simulink model "moore_mp3"  (R2024a)
settings: Solver=FixedStepDiscrete  StartTime=0.0  StopTime=inf  RelTol=1e-3  EnableMultiTasking=on
settings Model: Creator=nunkesser  LastModifiedBy=nunkesser
settings SolverCC: AlgebraicLoopSolver=TrustRegion
settings DataIOCC: LimitDataPoints=on  SaveFormat=Array  ReturnWorkspaceOutputs=off
settings OptimizationCC: LifeSpan=inf
settings DebuggingCC: SolverPrmCheckMsg=warning  UnconnectedInputMsg=warning  UnconnectedOutputMsg=warning  UnconnectedLineMsg=warning  SFUnexpectedBacktrackingDiag=warning  SFNoUnconditionalDefaultTransitionDiag=warning  SFExecutionAtInitializationDiag=none  ArithmeticOperatorsInVariantConditions=warning
settings HardwareCC: ProdBitPerPointer=32  ProdBitPerSizeT=32  ProdBitPerPtrDiffT=32  ProdLargestAtomicFloat=None  ProdIntDivRoundTo=Undefined  ProdEndianess=Unspecified  ProdWordSize=32  ProdHWDeviceType=32-bit Generic
settings ModelReferenceCC: PropagateSignalLabelsOutOfModel=off
settings SFSimCC: SimUseLocalCustomCode=off  CustomCodeUndefinedFunction=UseInterfaceOnly
settings RTWCC: RTWUseLocalCustomCode=off  GPUComputeCapability=3.5
settings CodeAppCC: StateflowObjectComments=on
settings GRTTargetCC: TargetLangStandard=C89/C90 (ANSI)
settings ConfigComp: CovMetricSettings=dw  CovSaveCumulativeToWorkspaceVar=on  CovSaveSingleToWorkspaceVar=on  CovExternalEMLEnable=off  CovSFcnEnable=off

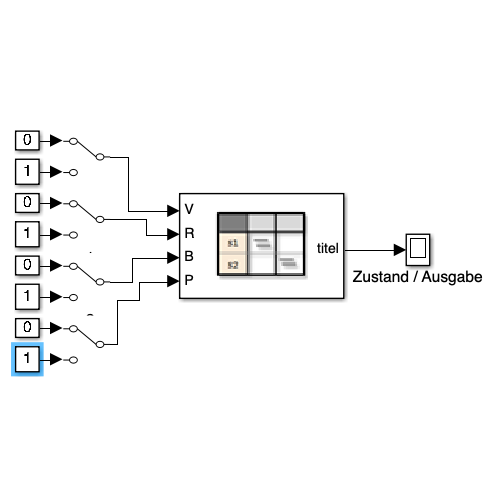
[thumbnail: Simulink's stored preview of the top-level diagram]
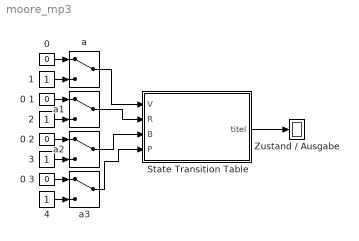
== system moore_mp3 ==
  0 {,1..3} (4 alike) : Constant  Value=0  OutDataTypeStr=boolean
  {1..4} (4 alike) : Constant  OutDataTypeStr=boolean
  State Transition Table : State Transition Table  TreatAsAtomicUnit=on
  Zustand / Ausgabe : Display
  a{,1..3} (4 alike) : ManualSwitch
  wires:
  1/1 -> a/2
  "0 "/1 -> a/1
  a/1 -> State Transition Table/1(V)
  2/1 -> a1/2
  0 1/1 -> a1/1
  a1/1 -> State Transition Table/2(R)
  3/1 -> a2/2
  0 2/1 -> a2/1
  a2/1 -> State Transition Table/3(B)
  4/1 -> a3/2
  0 3/1 -> a3/1
  a3/1 -> State Transition Table/4(P)
  State Transition Table/1(titel) -> Zustand / Ausgabe/1

== stateflow chart moore_mp3/State Transition Table ==
  state READY
    entry: titel=0
  state PLAY_TITLE_1
    entry: titel=1
  state PLAY_TITLE_2
    entry: titel=2
  state PLAY_TITLE_3
    entry: titel=3
  READY -> (junction 20) [order 2] : [P==0]
  (default) -> READY
  (junction 20) -> READY
  (junction 37) -> READY
  (junction 39) -> (junction 37)
  READY -> PLAY_TITLE_1 [order 1] : [P==1]
  PLAY_TITLE_1 -> READY [order 1] : [P==1]
  PLAY_TITLE_1 -> (junction 25) [order 2] : [(P==0) && (V==0) && (R==0) && (B==0)]
  (junction 25) -> PLAY_TITLE_1
  (junction 54) -> PLAY_TITLE_1
  (junction 56) -> (junction 54)
  PLAY_TITLE_1 -> (junction 61) [order 4] : [R==1]
  (junction 61) -> (junction 59)
  PLAY_TITLE_1 -> PLAY_TITLE_2 [order 3] : [V==1]
  PLAY_TITLE_1 -> PLAY_TITLE_2 [order 5] : [B==1]
  PLAY_TITLE_2 -> PLAY_TITLE_1 [order 4] : [R==1]
  PLAY_TITLE_2 -> (junction 45) [order 2] : [(P==0) && (V==0) && (R==0) && (B==0)]
  (junction 45) -> PLAY_TITLE_2
  PLAY_TITLE_2 -> (junction 39) [order 1] : [P==1]
  (junction 42) -> (junction 39)
  PLAY_TITLE_2 -> PLAY_TITLE_3 [order 3] : [V==1]
  PLAY_TITLE_2 -> PLAY_TITLE_3 [order 5] : [B==1]
  PLAY_TITLE_3 -> PLAY_TITLE_2 [order 4] : [R==1]
  PLAY_TITLE_3 -> (junction 48) [order 2] : [(P==0) && (V==0) && (R==0) && (B==0)]
  (junction 48) -> PLAY_TITLE_3
  PLAY_TITLE_3 -> (junction 42) [order 1] : [P==1]
  PLAY_TITLE_3 -> (junction 56) [order 3] : [V==1]
  (junction 59) -> PLAY_TITLE_3
  (junction 88) -> (junction 56)
  PLAY_TITLE_3 -> (junction 88) [order 5] : [B==1]
  data: titel output; V input; R input; B input; P input
